simulink model "threeAxisAttitudeControl"  (R2020b)
settings: Solver=VariableStepAuto  StartTime=0.0  StopTime=300  RelTol=1e-3
undefined symbols (not defined in the file): Angle, Axis, WMM2020
libraries: vrlib x3, robotcorelib x2, aerolibutil x2, aerolibgravity2 x1
settings Model: Creator=phill  LastModifiedBy=trave

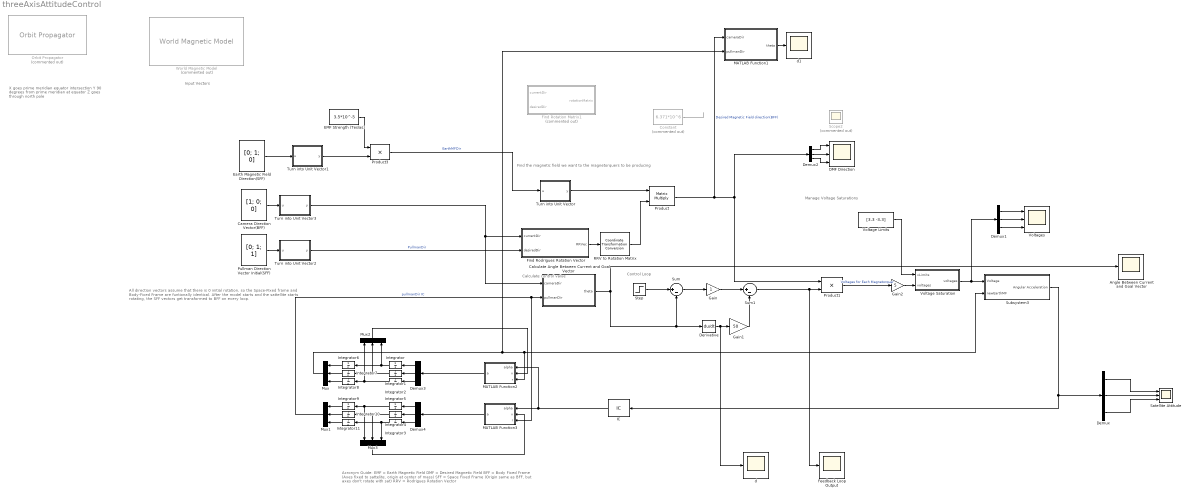
== system threeAxisAttitudeControl ==
  note: Calculate control value
  note: Manage Voltage Saturations
  note: Find the magnetic field we want to the magnetorquers to be producing
  note: Control Loop
  note: Input Vectors
  note: All direction vectors assume that there is 0 initial rotation, so the Space-FIxed frame and Body-Fixed Frame are funtionally identical. After the model starts and the sattellite starts rotating, the SFF vectors get transformed to BFF on every loop.
  note: X goes prime meridian equator intersection
      | Y 90 degrees from prime meridian at equator
      | Z goes through north pole
  note: Acronym Guide:
      | EMF = Earth Magnetic Field
      | DMF = Desired Magnetic Field
      | BFF = Body Fixed Frame (Axes fixed to sattelite, origin at center of mass)
      | SFF = Space Fixed Frame (Origin same as BFF, but axes don't rotate with sat)
      | RRV = Rodrigues Rotation Vector
  Angle Between Current and Goal Vector : Scope
  Calculate Angle Between Current and Goal Vector : MATLAB Function  TreatAsAtomicUnit=on
  Camera Direction Vector(BFF) : Constant  Value=[1; 0; 0]  VectorParams1D=off
  Constant : Constant  Commented=on  Value=6.371*10^6
  DMF Direction : Scope  NumInputPorts=3
  Demux{,1..4} (5 alike) : Demux  Outputs=3
  Derivative : Derivative
  EMF Strength (Teslas) : Constant  Value=3.5*10^-5
  Earth Magnetic Field Direction(SFF) : Constant  Value=[0; 1; 0]  VectorParams1D=off
  Feedback Loop Output : Scope
  Find Rodrigues Rotation Vector : MATLAB Function  TreatAsAtomicUnit=on
  Find Rotation Matrix1 : MATLAB Function  Commented=on  TreatAsAtomicUnit=on
  Gain : Gain
  Gain1 : Gain  Gain=50
  Gain2 : Gain  Gain=5
  IC : InitialCondition  Value=[0; 0; 0]
  Integrator{,1..6,8..9} (9 alike) : Integrator
  Integrator10 : Integrator  InitialCondition=1
  Integrator11 : Integrator  InitialCondition=1
  Integrator7 : Integrator  InitialCondition=1
  MATLAB Function1 : MATLAB Function  TreatAsAtomicUnit=on
  MATLAB Function2 : MATLAB Function  TreatAsAtomicUnit=on
  MATLAB Function3 : MATLAB Function  TreatAsAtomicUnit=on
  Mux{,1..3} (4 alike) : Mux  Inputs=3
  Orbit Propagator : OrbitPropagator  Commented=on  propagator=Numerical (high precision)  outportFrame=Fixed-frame  semiMajorAxis=6771.907  eccentricity=.00103  inclination=51.6  raan=244.3  argPeriapsis=353.735  trueAnomaly=199.683  customMu=4.305e13  customJ2=1.0826269e-03
      settings: AttributesFormatString=%<propagator>
  Product : Product  Multiplication=Matrix(*)
  Product1 : Product
  Product3 : Product
  Pullman Direction Vector Initial(SFF) : Constant  Value=[0; 1; 1]  VectorParams1D=off
  RRV to Rotation Matrix : robotcorelib/Coordinate Transformation Conversion  InputRepresentation=Axis-Angle  InputEulerSequence=ZYX  ShowTrVecInputPort=on  OutputRepresentation=Rotation Matrix  OutputEulerSequence=ZYX  ShowTrVecOutputPort=on  SimulateUsing=Interpreted execution
      settings: SourceProductBaseCode=NV,RO,RR,UV
  Satellite Attitude : Scope  NumInputPorts=3
  Scope2 : Scope  Commented=on
  Step : Step  After=0  SampleTime=0
  Subsystem3 : Subsystem
  Sum : Sum  Inputs=|+-
  Sum1 : Sum  Inputs=|+-
  Turn into Unit Vector : MATLAB Function  TreatAsAtomicUnit=on
  Turn into Unit Vector1 : MATLAB Function  TreatAsAtomicUnit=on
  Turn into Unit Vector2 : MATLAB Function  TreatAsAtomicUnit=on
  Turn into Unit Vector3 : MATLAB Function  TreatAsAtomicUnit=on
  Voltage Limits : Constant  Value=[3.3 -3.3]  VectorParams1D=off
  Voltage Saturation : MATLAB Function  TreatAsAtomicUnit=on
  Voltages : Scope  NumInputPorts=3
  World Magnetic Model : aerolibgravity2/World Magnetic Model  Commented=on  model=WMM2020 (2020-2025)  customFile='WMM2020.COF'  units=Metric (MKS)  time_in=on  month=January  day=1  year=2020  action=Error  h_out=on  dec_out=on  inc_out=on  ti_out=on
      settings: SourceProductBaseCode=AE
  d : Scope
  d1 : Scope
  wires:
  Find Rodrigues Rotation Vector/1(RRVec) -> RRV to Rotation Matrix/1
  Constant/1 -> ?
  Product/1 -> MATLAB Function1/1(cameraDir), Demux2/1, Product1/1  "Desired Magnetic Field direction(BFF)"
  Mux1/1 -> MATLAB Function3/3(r), Calculate Angle Between Current and Goal Vector/2(pullmanDir)  "pullmanDir IC"
  Calculate Angle Between Current and Goal Vector/1(theta) -> Derivative/1, Sum/2, Angle Between Current and Goal Vector/1
  Step/1 -> Sum/1
  Sum/1 -> Gain/1
  Gain/1 -> Sum1/1
  Derivative/1 -> d/1, Gain1/1
  Sum1/1 -> Feedback Loop Output/1, Product1/2
  Product1/1 -> Gain2/1  "Voltages for Each Magnetorquer"
  Subsystem3/1(Angular Acceleration) -> Demux/1, IC/1
  Demux/1 -> Satellite Attitude/1
  Demux/2 -> Satellite Attitude/2
  Demux/3 -> Satellite Attitude/3
  Voltage Saturation/1(voltages) -> Demux1/1, Subsystem3/1(Voltage)
  Voltage Limits/1 -> Voltage Saturation/1(vLimits)
  Demux1/1 -> Voltages/1
  Demux1/2 -> Voltages/2
  Demux1/3 -> Voltages/3
  Earth Magnetic Field Direction(SFF)/1 -> Turn into Unit Vector1/1(u)
  Turn into Unit Vector/1(y) -> Product/1
  EMF Strength (Teslas)/1 -> Product3/1
  Demux2/1 -> DMF Direction/1
  Demux2/2 -> DMF Direction/2
  Demux2/3 -> DMF Direction/3
  Product3/1 -> Turn into Unit Vector/1(u)  "EarthMFDir"
  RRV to Rotation Matrix/1 -> Product/2
  Gain1/1 -> Sum1/2
  Pullman Direction Vector Initial(SFF)/1 -> Turn into Unit Vector2/1(u)
  Camera Direction Vector(BFF)/1 -> Turn into Unit Vector3/1(u)
  Gain2/1 -> Voltage Saturation/2("voltages ")
  MATLAB Function1/1(theta) -> d1/1
  Turn into Unit Vector1/1(y) -> Product3/2
  Turn into Unit Vector3/1(y) -> Find Rodrigues Rotation Vector/1(currentDir), Calculate Angle Between Current and Goal Vector/1(cameraDir)
  Turn into Unit Vector2/1(y) -> Find Rodrigues Rotation Vector/2(desiredDir)  "PullmanDir"
  MATLAB Function2/1(a) -> Demux3/1
  MATLAB Function3/1(a) -> Demux4/1
  IC/1 -> MATLAB Function3/1(alpha), MATLAB Function2/1(alpha)
  Demux3/3 -> Integrator2/1
  Demux3/2 -> Integrator1/1
  Demux3/1 -> Integrator/1
  Demux4/1 -> Integrator5/1
  Demux4/2 -> Integrator4/1
  Demux4/3 -> Integrator3/1
  Integrator/1 -> Integrator6/1, Mux2/3
  Integrator1/1 -> Integrator7/1, Mux2/2
  Integrator2/1 -> Mux2/1, Integrator8/1
  Integrator5/1 -> Integrator9/1, Mux3/1
  Integrator4/1 -> Mux3/2, Integrator10/1
  Integrator3/1 -> Integrator11/1, Mux3/3
  Integrator6/1 -> Mux/1
  Integrator7/1 -> Mux/2
  Integrator8/1 -> Mux/3
  Integrator9/1 -> Mux1/1
  Integrator10/1 -> Mux1/2
  Integrator11/1 -> Mux1/3
  Mux/1 -> Subsystem3/2(newEarthMF), MATLAB Function2/3(r), MATLAB Function1/2(pullmanDir)
  Mux2/1 -> MATLAB Function2/2(v)
  Mux3/1 -> MATLAB Function3/2(v)

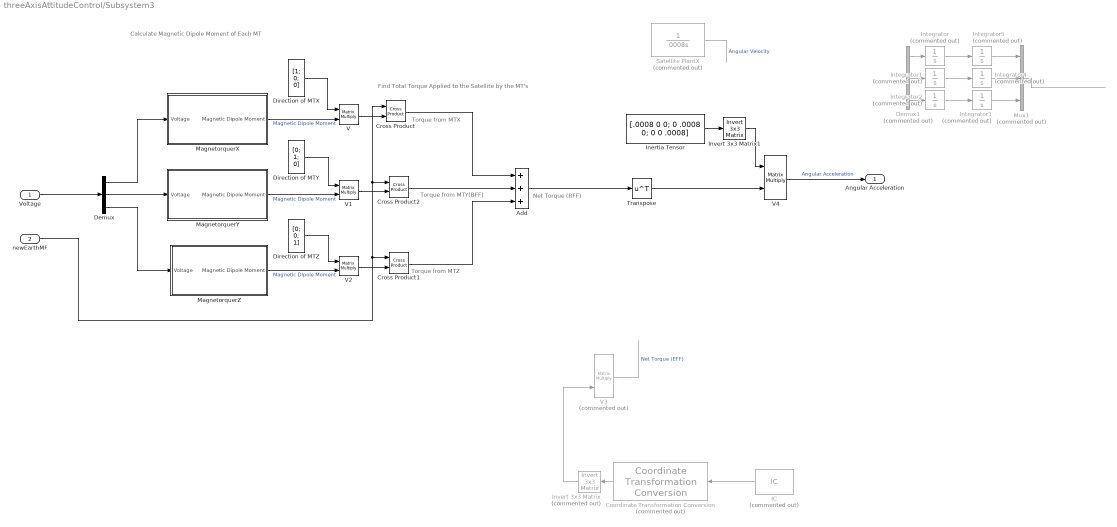
== system threeAxisAttitudeControl/Subsystem3 ==
  note: Find Total Torque Applied to the Satellite by the MT's
  note: Calculate Magnetic Dipole Moment of Each MT
  note: Net Torque (BFF)
  note: Torque from MTZ
  note: Torque from MTX
  note: Torque from MTY(BFF)
  Voltage : Inport
  newEarthMF : Inport  Port=2
  Add : Sum  Inputs=+++
  Coordinate Transformation Conversion : robotcorelib/Coordinate Transformation Conversion  Commented=on  InputRepresentation=Euler Angles  InputEulerSequence=XYZ  ShowTrVecInputPort=on  OutputRepresentation=Rotation Matrix  OutputEulerSequence=ZYX  ShowTrVecOutputPort=on  SimulateUsing=Interpreted execution
      settings: SourceProductBaseCode=NV,RO,RR,UV
  Cross Product : vrlib/Utilities/Cross Product
  Cross Product1 : vrlib/Utilities/Cross Product
  Cross Product2 : vrlib/Utilities/Cross Product
  Demux : Demux  Outputs=3
  Demux1 : Demux  Commented=on  Outputs=3
  Direction of MTX : Constant  Value=[1; 0; 0]  VectorParams1D=off
  Direction of MTY : Constant  Value=[0; 1; 0]  VectorParams1D=off
  Direction of MTZ : Constant  Value=[0; 0; 1]  VectorParams1D=off
  IC : InitialCondition  Commented=on  Value=[0 0 0]
  Inertia Tensor : Constant  Value=[.0008 0 0; 0 .0008 0; 0 0 .0008]
  Integrator{,1..5} (6 alike) : Integrator  Commented=on
  Invert 3x3 Matrix : aerolibutil/Invert  3x3 Matrix  Commented=on
  Invert 3x3 Matrix1 : aerolibutil/Invert  3x3 Matrix
  MagnetorquerX : Subsystem
  MagnetorquerY : Subsystem
  MagnetorquerZ : Subsystem
  Mux1 : Mux  Commented=on  Inputs=3
  Satellite PlantX : TransferFcn  Commented=on  Denominator=[.0008 0]
  Transpose : Math  Operator=transpose  SaturateOnIntegerOverflow=on
  V{,1..2,4} (4 alike) : Product  Multiplication=Matrix(*)
  V3 : Product  Commented=on  Multiplication=Matrix(*)
  Angular Acceleration : Outport
  wires:
  Cross Product1/1 -> Add/3
  Cross Product/1 -> Add/1
  Cross Product2/1 -> Add/2
  MagnetorquerZ/1(Magnetic Dipole Moment) -> V2/2  "Magnetic Dipole Moment"
  MagnetorquerY/1(Magnetic Dipole Moment) -> V1/2  "Magnetic Dipole Moment"
  Demux/1 -> MagnetorquerX/1(Voltage)
  Demux/2 -> MagnetorquerY/1(Voltage)
  MagnetorquerX/1(Magnetic Dipole Moment) -> V/2  "Magnetic Dipole Moment"
  Satellite PlantX/1 -> ?  "Angular Velocity"
  Demux/3 -> MagnetorquerZ/1(Voltage)
  newEarthMF/1 -> Cross Product/1, Cross Product2/1, Cross Product1/1
  Direction of MTZ/1 -> V2/1
  Direction of MTY/1 -> V1/1
  Direction of MTX/1 -> V/1
  V/1 -> Cross Product/2
  V1/1 -> Cross Product2/2
  V2/1 -> Cross Product1/2
  Coordinate Transformation Conversion/1 -> Invert 3x3 Matrix/1
  Invert 3x3 Matrix/1 -> V3/2
  Inertia Tensor/1 -> Invert 3x3 Matrix1/1
  Invert 3x3 Matrix1/1 -> V4/1
  V3/1 -> ?  "Net Torque (EFF)"
  IC/1 -> Coordinate Transformation Conversion/1
  Add/1 -> Transpose/1
  Transpose/1 -> V4/2
  Demux1/3 -> Integrator2/1
  Integrator3/1 -> Mux1/3
  Mux1/1 -> ?
  Integrator5/1 -> Mux1/1
  Integrator2/1 -> Integrator3/1
  Demux1/2 -> Integrator1/1
  Integrator/1 -> Integrator5/1
  Integrator1/1 -> Integrator4/1
  Demux1/1 -> Integrator/1
  Integrator4/1 -> Mux1/2
  V4/1 -> Angular Acceleration/1  "Angular Acceleration"
  Voltage/1 -> Demux/1

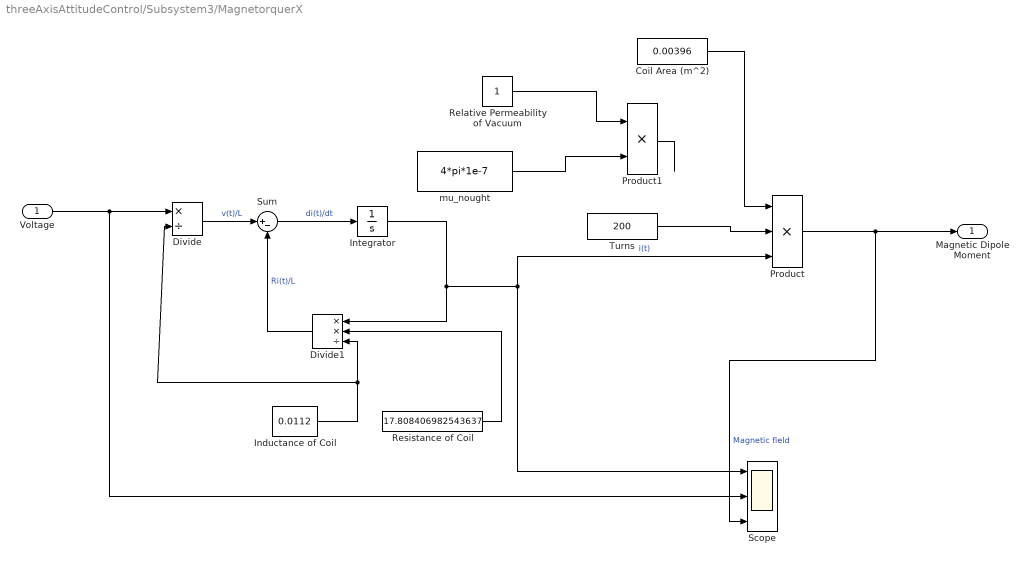
== system threeAxisAttitudeControl/Subsystem3/MagnetorquerX ==
  Voltage : Inport
  Coil Area (m^2) : Constant  Value=0.00396
  Divide : Product  Inputs=*/
  Divide1 : Product  Inputs=**/
  Inductance of Coil : Constant  Value=0.0112
  Integrator : Integrator
  Product : Product  Inputs=3
  Product1 : Product
  Relative Permeability of Vacuum : Constant
  "Resistance of Coil " : Constant  Value=17.808406982543637
  Scope : Scope  NumInputPorts=3
  Sum : Sum  Inputs=|+-
  Turns : Constant  Value=200
  mu_nought : Constant  Value=4*pi*1e-7
  Magnetic Dipole Moment : Outport  VectorParamsAs1DForOutWhenUnconnected=off
  wires:
  Sum/1 -> Integrator/1  "di(t)/dt"
  "Resistance of Coil "/1 -> Divide1/2
  Inductance of Coil/1 -> Divide1/3, Divide/2
  Divide/1 -> Sum/1  "v(t)/L"
  Integrator/1 -> Product/3, Scope/1, Divide1/1  "i(t)"
  Divide1/1 -> Sum/2  "Ri(t)/L"
  Coil Area (m^2)/1 -> Product/1
  Turns/1 -> Product/2
  Product/1 -> Magnetic Dipole Moment/1, Scope/3  "Magnetic field"
  Voltage/1 -> Scope/2, Divide/1
  Relative Permeability of Vacuum/1 -> Product1/1
  mu_nought/1 -> Product1/2
  Product1/1 -> ?

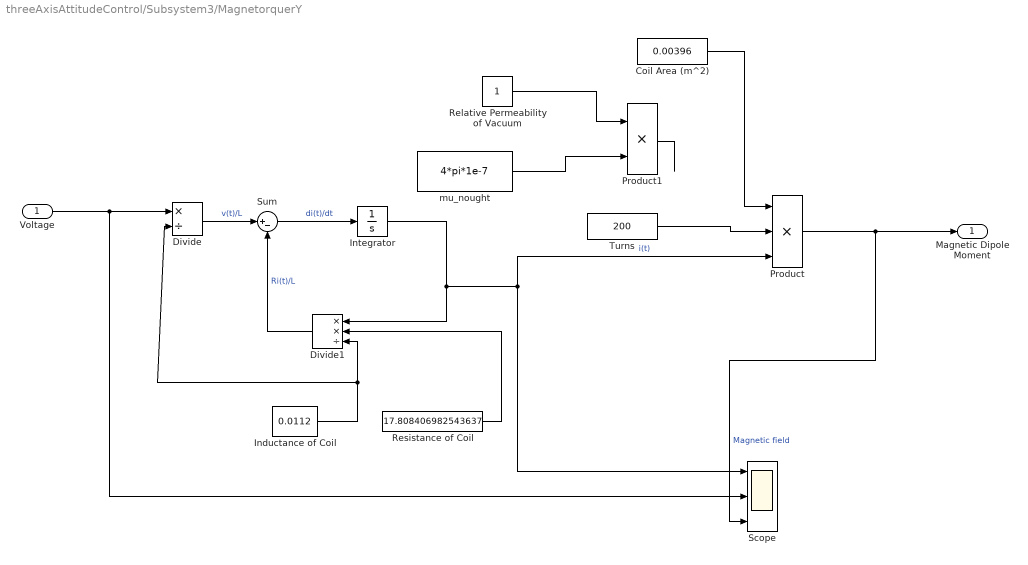
== system threeAxisAttitudeControl/Subsystem3/MagnetorquerY ==
  Voltage : Inport
  Coil Area (m^2) : Constant  Value=0.00396
  Divide : Product  Inputs=*/
  Divide1 : Product  Inputs=**/
  Inductance of Coil : Constant  Value=0.0112
  Integrator : Integrator
  Product : Product  Inputs=3
  Product1 : Product
  Relative Permeability of Vacuum : Constant
  "Resistance of Coil " : Constant  Value=17.808406982543637
  Scope : Scope  NumInputPorts=3
  Sum : Sum  Inputs=|+-
  Turns : Constant  Value=200
  mu_nought : Constant  Value=4*pi*1e-7
  Magnetic Dipole Moment : Outport  VectorParamsAs1DForOutWhenUnconnected=off
  wires:
  Sum/1 -> Integrator/1  "di(t)/dt"
  "Resistance of Coil "/1 -> Divide1/2
  Inductance of Coil/1 -> Divide1/3, Divide/2
  Divide/1 -> Sum/1  "v(t)/L"
  Integrator/1 -> Product/3, Scope/1, Divide1/1  "i(t)"
  Divide1/1 -> Sum/2  "Ri(t)/L"
  Coil Area (m^2)/1 -> Product/1
  Turns/1 -> Product/2
  Product/1 -> Magnetic Dipole Moment/1, Scope/3  "Magnetic field"
  Voltage/1 -> Scope/2, Divide/1
  Relative Permeability of Vacuum/1 -> Product1/1
  mu_nought/1 -> Product1/2
  Product1/1 -> ?

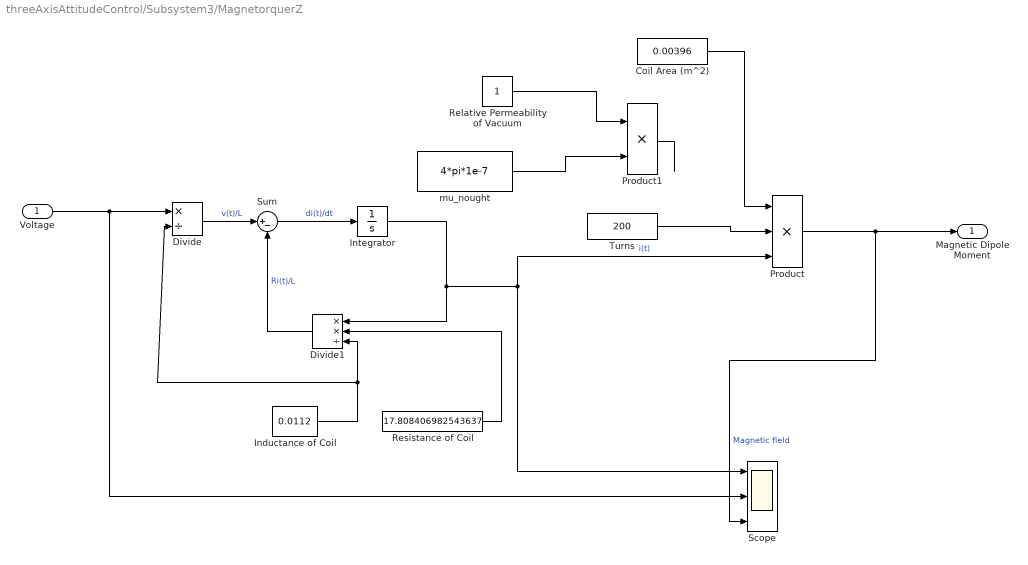
== system threeAxisAttitudeControl/Subsystem3/MagnetorquerZ ==
  Voltage : Inport
  Coil Area (m^2) : Constant  Value=0.00396
  Divide : Product  Inputs=*/
  Divide1 : Product  Inputs=**/
  Inductance of Coil : Constant  Value=0.0112
  Integrator : Integrator
  Product : Product  Inputs=3
  Product1 : Product
  Relative Permeability of Vacuum : Constant
  "Resistance of Coil " : Constant  Value=17.808406982543637
  Scope : Scope  NumInputPorts=3
  Sum : Sum  Inputs=|+-
  Turns : Constant  Value=200
  mu_nought : Constant  Value=4*pi*1e-7
  Magnetic Dipole Moment : Outport  VectorParamsAs1DForOutWhenUnconnected=off
  wires:
  Sum/1 -> Integrator/1  "di(t)/dt"
  "Resistance of Coil "/1 -> Divide1/2
  Inductance of Coil/1 -> Divide1/3, Divide/2
  Divide/1 -> Sum/1  "v(t)/L"
  Integrator/1 -> Product/3, Scope/1, Divide1/1  "i(t)"
  Divide1/1 -> Sum/2  "Ri(t)/L"
  Coil Area (m^2)/1 -> Product/1
  Turns/1 -> Product/2
  Product/1 -> Magnetic Dipole Moment/1, Scope/3  "Magnetic field"
  Voltage/1 -> Scope/2, Divide/1
  Relative Permeability of Vacuum/1 -> Product1/1
  mu_nought/1 -> Product1/2
  Product1/1 -> ?

== matlab function threeAxisAttitudeControl/Find Rodrigues Rotation Vector ==
  data: currentDir input; RRVec output; desiredDir input
function RRVec = fcn(currentDir, desiredDir)
% #codegen

RRVec = [0; 0; 0; 0]; % initialize Rodriguez Rotation vector

% find axis of rotation
crossProduct = cross(currentDir, desiredDir);
RRVec(1:3) = crossProduct / norm(crossProduct); % 

% find angle of rotation
dotProduct = dot(desiredDir, currentDir);
RRVec(4) = acos(dotProduct);

== matlab function threeAxisAttitudeControl/MATLAB Function3 ==
  data: alpha input; a output; v input; r input
function a = fcn(alpha, v, r)
% make everything into column vectors because simulink will change them
% sometimes for some reason
alpha = [alpha(1); alpha(2); alpha(3)];
v = [v(1); v(2); v(3)];
r = [r(1); r(2); r(3)];


% acceleration of point r tangent to its rotation
aTangent = cross(alpha, r);

% radial acceleration from centrifugal force
rMag = sqrt(dot(r,r));
aRadial = (dot(v,v) / rMag) * (-1 * (r / rMag));

% acceleration of point r
a = aRadial + aTangent;

== matlab function threeAxisAttitudeControl/Calculate Angle Between Current and Goal Vector ==
  data: cameraDir input; pullmanDir input; theta output
function theta = fcn(cameraDir, pullmanDir)
% #codegen
mag = norm(cameraDir)*norm(pullmanDir);
if mag == 0
    theta = pi/2;
else
    x = dot(cameraDir, pullmanDir) / mag;

    theta = acos(x);
end

== matlab function threeAxisAttitudeControl/Voltage Saturation ==
  data: vLimits input; voltages output; voltages input
function voltages = fcn(vLimits, voltages)
for i = 1:3
   if voltages(i) > vLimits(1)
       voltages = voltages * (vLimits(1) / voltages(i));
   elseif voltages(i) < vLimits(2)
       voltages = voltages * (vLimits(2) / voltages(i));
   end
end

== matlab function threeAxisAttitudeControl/Find Rotation Matrix1 ==
  data: currentDir input; rotationMatrix output; desiredDir input
function rotationMatrix = fcn(currentDir, desiredDir)
% #codegen

RRVec = [0 0 0 0]; % initialize Rodriguez Rotation vector

% find axis of rotation
crossProduct = cross(desiredDir, currentDir);
RRVec(1:3) = crossProduct / norm(crossProduct); % 

% find angle of rotation
dotProduct = dot(desiredDir, currentDir);
RRVec(4) = acos(dotProduct);

matrix = zeros(3);


phi = RRVec(4);
u = RRVec(1);
v = RRVec(2);
w = RRVec(3);

% internet code. Gooes from Rodrigues Rotation vector to rotation matrix

rcos = cos(phi);
rsin = sin(phi);
matrix(1,1) =      rcos + u*u*(1-rcos);
matrix(2,1) =  w * rsin + v*u*(1-rcos);
matrix(1,3) = -v * rsin + w*u*(1-rcos);
matrix(2,1) = -w * rsin + u*v*(1-rcos);
matrix(2,2) =      rcos + v*v*(1-rcos);
matrix(2,3) =  u * rsin + w*v*(1-rcos);
matrix(3,1) =  v * rsin + u*w*(1-rcos);
matrix(3,2) = -u * rsin + v*w*(1-rcos);
matrix(3,3) =      rcos + w*w*(1-rcos);

rotationMatrix = matrix;

== matlab function threeAxisAttitudeControl/Turn into Unit Vector1 ==
  data: u input; y output
function y = fcn(u)
% #codegen

mag = norm(u);

y = (u/mag);

== matlab function threeAxisAttitudeControl/MATLAB Function1 ==
  data: cameraDir input; pullmanDir input; theta output
function theta = fcn(cameraDir, pullmanDir)
% #codegen
x = dot(cameraDir, pullmanDir) / (norm(cameraDir)*norm(pullmanDir));

theta = acos(x);

== matlab function threeAxisAttitudeControl/Turn into Unit Vector2 ==
  data: u input; y output
function y = fcn(u)
% #codegen

mag = norm(u);

y = (u/mag);

== matlab function threeAxisAttitudeControl/Turn into Unit Vector3 ==
  data: u input; y output
function y = fcn(u)
% #codegen

mag = norm(u);

y = (u/mag);

== matlab function threeAxisAttitudeControl/MATLAB Function2 ==
  data: alpha input; a output; v input; r input
function a = fcn(alpha, v, r)
% make everything into column vectors because simulink will change them
% sometimes for some reason
alpha = [alpha(1); alpha(2); alpha(3)];
v = [v(1); v(2); v(3)];
r = [r(1); r(2); r(3)];


% acceleration of point r tangent to its rotation
aTangent = cross(alpha, r);

% radial acceleration from centrifugal force
rMag = sqrt(dot(r,r));
aRadial = (dot(v,v) / rMag) * (-1 * (r / rMag));

% acceleration of point r
a = aRadial + aTangent;

== matlab function threeAxisAttitudeControl/Turn into Unit Vector ==
  data: u input; y output
function y = fcn(u)
% #codegen

mag = norm(u);

y = (u/mag)';
